simulink model "three_level_sv"  (R2025a)
settings: Solver=ode1be  StartTime=0.0  StopTime=simlength  FixedStep=ts_sim  MaxStep=ts_sim
undefined symbols (not defined in the file): number_of_cells, Q, q1Kalman, q2Kalman, q3Kalman, rKalman, tc, ts_afe, ts_zvs, tsample, Vbattery_nom
libraries: fl_lib x59, nesl_utility x30, ee_lib x1, lithium_ion_cell_lib x1, simulink x1
(part 2 of 2)

== system three_level_sv/theee-level-inverter/three-level-inverter/stage-1/three-level-inverter/switch_3 ==
  Diode : fl_lib/Electrical/Electrical Elements/Diode  Vf=Vdon_diode V  Ron=Rdon_diode Ohm  Goff=1e-8 1/Ohm  i_specify=off  i_priority=None  i=0 A  i_nominal_specify=off  i_nominal_value=1  i_nominal_unit=A  v_specify=off  v_priority=None  v=0 V  v_nominal_specify=off  v_nominal_value=1  v_nominal_unit=V
  Switch : fl_lib/Electrical/Electrical Elements/Switch  R_closed=Ron Ohm  G_open=1e-8 1/Ohm  Threshold=7.5  i_specify=off  i_priority=None  i=0 A  i_nominal_specify=off  i_nominal_value=1  i_nominal_unit=A  v_specify=off  v_priority=None  v=0 V  v_nominal_specify=off  v_nominal_value=1  v_nominal_unit=V
  G : PMIOPort  Side=Left
  C : PMIOPort  Port=2  Side=Left
  E : PMIOPort  Port=3  Side=Right
  connections:
  Diode/LConn1 -- E/RConn1 -- Switch/LConn1
  Switch/RConn1 -- G/RConn1
  Switch/RConn2 -- Diode/RConn1 -- C/RConn1

== system three_level_sv/theee-level-inverter/three-level-inverter/stage-1/three-level-inverter/switch_4 ==
  Diode : fl_lib/Electrical/Electrical Elements/Diode  Vf=Vdon_diode V  Ron=Rdon_diode Ohm  Goff=1e-8 1/Ohm  i_specify=off  i_priority=None  i=0 A  i_nominal_specify=off  i_nominal_value=1  i_nominal_unit=A  v_specify=off  v_priority=None  v=0 V  v_nominal_specify=off  v_nominal_value=1  v_nominal_unit=V
  Switch : fl_lib/Electrical/Electrical Elements/Switch  R_closed=Ron Ohm  G_open=1e-8 1/Ohm  Threshold=7.5  i_specify=off  i_priority=None  i=0 A  i_nominal_specify=off  i_nominal_value=1  i_nominal_unit=A  v_specify=off  v_priority=None  v=0 V  v_nominal_specify=off  v_nominal_value=1  v_nominal_unit=V
  G : PMIOPort  Side=Left
  C : PMIOPort  Port=2  Side=Left
  E : PMIOPort  Port=3  Side=Right
  connections:
  C/RConn1 -- Diode/RConn1 -- Switch/RConn2
  Switch/RConn1 -- G/RConn1
  Switch/LConn1 -- E/RConn1 -- Diode/LConn1

== system three_level_sv/theee-level-inverter/three-level-inverter/stage-1/three-level-inverter/switch_5 ==
  Diode : fl_lib/Electrical/Electrical Elements/Diode  Vf=Vdon_diode V  Ron=Rdon_diode Ohm  Goff=1e-8 1/Ohm  i_specify=off  i_priority=None  i=0 A  i_nominal_specify=off  i_nominal_value=1  i_nominal_unit=A  v_specify=off  v_priority=None  v=0 V  v_nominal_specify=off  v_nominal_value=1  v_nominal_unit=V
  Switch : fl_lib/Electrical/Electrical Elements/Switch  R_closed=Ron Ohm  G_open=1e-8 1/Ohm  Threshold=7.5  i_specify=off  i_priority=None  i=0 A  i_nominal_specify=off  i_nominal_value=1  i_nominal_unit=A  v_specify=off  v_priority=None  v=0 V  v_nominal_specify=off  v_nominal_value=1  v_nominal_unit=V
  G : PMIOPort  Side=Left
  C : PMIOPort  Port=2  Side=Left
  E : PMIOPort  Port=3  Side=Right
  connections:
  Diode/LConn1 -- E/RConn1 -- Switch/LConn1
  Switch/RConn1 -- G/RConn1
  Switch/RConn2 -- Diode/RConn1 -- C/RConn1

== system three_level_sv/theee-level-inverter/three-level-inverter/stage-1/three-level-inverter/switch_6 ==
  Diode : fl_lib/Electrical/Electrical Elements/Diode  Vf=Vdon_diode V  Ron=Rdon_diode Ohm  Goff=1e-8 1/Ohm  i_specify=off  i_priority=None  i=0 A  i_nominal_specify=off  i_nominal_value=1  i_nominal_unit=A  v_specify=off  v_priority=None  v=0 V  v_nominal_specify=off  v_nominal_value=1  v_nominal_unit=V
  Switch : fl_lib/Electrical/Electrical Elements/Switch  R_closed=Ron Ohm  G_open=1e-8 1/Ohm  Threshold=7.5  i_specify=off  i_priority=None  i=0 A  i_nominal_specify=off  i_nominal_value=1  i_nominal_unit=A  v_specify=off  v_priority=None  v=0 V  v_nominal_specify=off  v_nominal_value=1  v_nominal_unit=V
  G : PMIOPort  Side=Left
  C : PMIOPort  Port=2  Side=Left
  E : PMIOPort  Port=3  Side=Right
  connections:
  C/RConn1 -- Diode/RConn1 -- Switch/RConn2
  Switch/RConn1 -- G/RConn1
  Switch/LConn1 -- E/RConn1 -- Diode/LConn1

== system three_level_sv/theee-level-inverter/three-level-inverter/stage-1/three-level-inverter/switch_7 ==
  Diode : fl_lib/Electrical/Electrical Elements/Diode  Vf=Vdon_diode V  Ron=Rdon_diode Ohm  Goff=1e-8 1/Ohm  i_specify=off  i_priority=None  i=0 A  i_nominal_specify=off  i_nominal_value=1  i_nominal_unit=A  v_specify=off  v_priority=None  v=0 V  v_nominal_specify=off  v_nominal_value=1  v_nominal_unit=V
  Switch : fl_lib/Electrical/Electrical Elements/Switch  R_closed=Ron Ohm  G_open=1e-8 1/Ohm  Threshold=7.5  i_specify=off  i_priority=None  i=0 A  i_nominal_specify=off  i_nominal_value=1  i_nominal_unit=A  v_specify=off  v_priority=None  v=0 V  v_nominal_specify=off  v_nominal_value=1  v_nominal_unit=V
  G : PMIOPort  Side=Left
  C : PMIOPort  Port=2  Side=Left
  E : PMIOPort  Port=3  Side=Right
  connections:
  Diode/LConn1 -- E/RConn1 -- Switch/LConn1
  Switch/RConn1 -- G/RConn1
  Switch/RConn2 -- Diode/RConn1 -- C/RConn1

== system three_level_sv/theee-level-inverter/three-level-inverter/stage-1/three-level-inverter/switch_8 ==
  Diode : fl_lib/Electrical/Electrical Elements/Diode  Vf=Vdon_diode V  Ron=Rdon_diode Ohm  Goff=1e-8 1/Ohm  i_specify=off  i_priority=None  i=0 A  i_nominal_specify=off  i_nominal_value=1  i_nominal_unit=A  v_specify=off  v_priority=None  v=0 V  v_nominal_specify=off  v_nominal_value=1  v_nominal_unit=V
  Switch : fl_lib/Electrical/Electrical Elements/Switch  R_closed=Ron Ohm  G_open=1e-8 1/Ohm  Threshold=7.5  i_specify=off  i_priority=None  i=0 A  i_nominal_specify=off  i_nominal_value=1  i_nominal_unit=A  v_specify=off  v_priority=None  v=0 V  v_nominal_specify=off  v_nominal_value=1  v_nominal_unit=V
  G : PMIOPort  Side=Left
  C : PMIOPort  Port=2  Side=Left
  E : PMIOPort  Port=3  Side=Right
  connections:
  C/RConn1 -- Diode/RConn1 -- Switch/RConn2
  Switch/RConn1 -- G/RConn1
  Switch/LConn1 -- E/RConn1 -- Diode/LConn1

== system three_level_sv/theee-level-inverter/three-level-inverter/stage-1/three-level-inverter/switch_9 ==
  Diode : fl_lib/Electrical/Electrical Elements/Diode  Vf=Vdon_diode V  Ron=Rdon_diode Ohm  Goff=1e-8 1/Ohm  i_specify=off  i_priority=None  i=0 A  i_nominal_specify=off  i_nominal_value=1  i_nominal_unit=A  v_specify=off  v_priority=None  v=0 V  v_nominal_specify=off  v_nominal_value=1  v_nominal_unit=V
  Switch : fl_lib/Electrical/Electrical Elements/Switch  R_closed=Ron Ohm  G_open=1e-8 1/Ohm  Threshold=7.5  i_specify=off  i_priority=None  i=0 A  i_nominal_specify=off  i_nominal_value=1  i_nominal_unit=A  v_specify=off  v_priority=None  v=0 V  v_nominal_specify=off  v_nominal_value=1  v_nominal_unit=V
  G : PMIOPort  Side=Left
  C : PMIOPort  Port=2  Side=Left
  E : PMIOPort  Port=3  Side=Right
  connections:
  Diode/LConn1 -- E/RConn1 -- Switch/LConn1
  Switch/RConn1 -- G/RConn1
  Switch/RConn2 -- Diode/RConn1 -- C/RConn1

== matlab function three_level_sv/theee-level-inverter/pwm_commands/abc2alphabeta ==
  data: u input; alpha output; v input; w input; beta output
function [alpha,beta] = abc2alphabeta(u, v, w)

    alpha = 2/3 * (u - 1/2 * v - 1/2 * w);
    beta = 2/3 * (sqrt(3)/2 * v - sqrt(3)/2 * w);

end

== matlab function three_level_sv/theee-level-inverter/pwm_commands/counter_6 ==
  data: y output; Nmax parameter
function y = count_index(Nmax)

coder.extrinsic('evalin'); 

persistent x
    if isempty(x)
        x = 1;
    end

    if (x >= Nmax)
        x = 1;
    else
        x = x + 1;
    end


    if (x >= Nmax)
        y = Nmax;
    elseif (x <= 1)
        y = 1;
    else
        y = x;
    end
end

== matlab function three_level_sv/theee-level-inverter/pwm_commands/index2sv_6 ==
  data: i input; y output
function y = inner_sv_index(i)

    if (i == 1)
        y = [1 0 0]; 
    elseif (i == 2)
        y = [1 1 0]; 
    elseif (i == 3)
        y = [0 1 0]; 
    elseif (i == 4)
        y = [0 1 1]; 
    elseif (i == 5)
        y = [0 0 1];     
    elseif (i == 6)
        y = [1 0 1]; 
    else
        y = [0 0 0];
    end
end

== matlab function three_level_sv/theee-level-inverter/pwm_commands/index2sv_12 ==
  data: i input; y output
function y = outer_sv_index(i)

    if (i == 1)
        y = [1 -1 -1]; 
    elseif (i == 2)
        y = [1 0 -1]; 
    elseif (i == 3)
        y = [1 1 -1]; 
    elseif (i == 4)
        y = [0 1 -1]; 
    elseif (i == 5)
        y = [-1 1 -1];     
    elseif (i == 6)
        y = [-1 1 0]; 
    elseif (i == 7)
        y = [-1 1 1]; 
    elseif (i == 8)
        y = [-1 0 1]; 
    elseif (i == 9)
        y = [-1 -1 1]; 
    elseif (i == 10)
        y = [0 -1 1];
    elseif (i == 11)
        y = [1 -1 1]; 
    elseif (i == 12)
        y = [1 -1 0]; 
    else
        y = [0 0 0];
    end
end

== matlab function three_level_sv/theee-level-inverter/pwm_commands/sv2gata_cmds ==
  data: u input; y output
function y = three_level_sv(u)

u_nnn = [-1 -1 -1];
u_nno = [-1 -1 0];
u_nnp = [-1 -1 1];

u_non = [-1 0 -1];
u_noo = [-1 0 0];
u_nop = [-1 0 1];

u_npn = [-1 1 -1];
u_npo = [-1 1 0];
u_npp = [-1 1 1];

u_onn = [0 -1 -1];
u_ono = [0 -1 0];
u_onp = [0 -1 1];

u_oon = [0 0 -1];
u_ooo = [0 0 0];
u_oop = [0 0 1];

u_opn = [0 1 -1];
u_opo = [0 1 0];
u_opp = [0 1 1];

u_pnn = [1 -1 -1];
u_pno = [1 -1 0];
u_pnp = [1 -1 1];

u_pon = [1 0 -1];
u_poo = [1 0 0];
u_pop = [1 0 1];

u_ppn = [1 1 -1];
u_ppo = [1 1 0];
u_ppp = [1 1 1];

u_nnn_g = [0 0 1 1 0 0 1 1 0 0 1 1];
u_nno_g = [0 0 1 1 0 0 1 1 0 1 1 0];
u_nnp_g = [0 0 1 1 0 0 1 1 1 1 0 0];

u_non_g = [0 0 1 1 0 1 1 0 0 0 1 1];
u_noo_g = [0 0 1 1 0 1 1 0 0 1 1 0];
u_nop_g = [0 0 1 1 0 1 1 0 1 1 0 0];

u_npn_g = [0 0 1 1 1 1 0 0 0 0 1 1];
u_npo_g = [0 0 1 1 1 1 0 0 0 1 1 0];
u_npp_g = [0 0 1 1 1 1 0 0 1 1 0 0];

u_onn_g = [0 1 1 0 0 0 1 1 0 0 1 1];
u_ono_g = [0 1 1 0 0 0 1 1 0 1 1 0];
u_onp_g = [0 1 1 0 0 0 1 1 1 1 0 0];

u_oon_g = [0 1 1 0 0 1 1 0 0 0 1 1];
u_ooo_g = [0 1 1 0 0 1 1 0 0 1 1 0];
u_oop_g = [0 1 1 0 0 1 1 0 1 1 0 0];

u_opn_g = [0 1 1 0 1 1 0 0 0 0 1 1];
u_opo_g = [0 1 1 0 1 1 0 0 0 1 1 0];
u_opp_g = [0 1 1 0 1 1 0 0 1 1 0 0];

u_pnn_g = [1 1 0 0 0 0 1 1 0 0 1 1];
u_pno_g = [1 1 0 0 0 0 1 1 0 1 1 0];
u_pnp_g = [1 1 0 0 0 0 1 1 1 1 0 0];

u_pon_g = [1 1 0 0 0 1 1 0 0 0 1 1];
u_poo_g = [1 1 0 0 0 1 1 0 0 1 1 0];
u_pop_g = [1 1 0 0 0 1 1 0 1 1 0 0];

u_ppn_g = [1 1 0 0 1 1 0 0 0 0 1 1];
u_ppo_g = [1 1 0 0 1 1 0 0 0 1 1 0];
u_ppp_g = [1 1 0 0 1 1 0 0 1 1 0 0];

if (u == u_nnn)
y = u_nnn_g;
elseif (u == u_nno)
y = u_nno_g;
elseif (u == u_nnp)
y = u_nnp_g;
elseif (u == u_non)
y = u_non_g;
elseif (u == u_noo)
y = u_noo_g;
elseif (u == u_nop)
y = u_nop_g;
elseif (u == u_npn)
y = u_npn_g;
elseif (u == u_npo)
y = u_npo_g;
elseif (u == u_npp)
y = u_npp_g;
elseif (u == u_onn)
y = u_onn_g;
elseif (u == u_ono)
y = u_ono_g;
elseif (u == u_onp)
y = u_onp_g;
elseif (u == u_oon)
y = u_oon_g;
elseif (u == u_ooo)
y = u_ooo_g;
elseif (u == u_oop)
y = u_oop_g;
elseif (u == u_opn)
y = u_opn_g;
elseif (u == u_opo)
y = u_opo_g;
elseif (u == u_opp)
y = u_opp_g;
elseif (u == u_pnn)
y = u_pnn_g;
elseif (u == u_pno)
y = u_pno_g;
elseif (u == u_pnp)
y = u_pnp_g;
elseif (u == u_pon)
y = u_pon_g;
elseif (u == u_poo)
y = u_poo_g;
elseif (u == u_pop)
y = u_pop_g;
elseif (u == u_ppn)
y = u_ppn_g;
elseif (u == u_ppo)
y = u_ppo_g;
elseif (u == u_ppp)
y = u_ppp_g;
else
   y = u_ooo_g; 
end

== matlab function three_level_sv/theee-level-inverter/battery_system/LithiumIonBattery/SOC_estimator/Kalman_observer/kalman_observer_gains ==
  data: i input; ts input; l1 output; z input; q1 input; q2 input; q3 input; r input; Q input; l2 output; l3 output
function [l1,l2,l3] = EKF(i,ts,z,q1,q2,q3,r,Q)

    persistent  p11 p12 p13 p21 p22 p23 p31 p32 p33

    if isempty(p11)
        p11 = q1;
        p12 = 0;
        p13 = 0;
        p21 = 0;
        p22 = q2;
        p23 = 0;
        p31 = 0;
        p32 = 0;
        p33 = q3;
    end
    R = 0.15;
    C = 10;
    M = 125;
    E_1 = -1.031;
    E1 = 0.2156;
    E2 = 0;
    E3 = 0;
    Elog = -0.05;
    alpha = 35;

    a11 = 1;
    a12 = 0;
    a13 = 0;
    a21 = 0;
    a22 = exp(-ts/(R*C));
    a23 = 0;
    a31 = 0;
    a32 = 0;
    a33 = abs(exp(-i*ts/Q));

    c1 = -alpha*E_1*abs(exp(-alpha*z)) + E1 + 2*E2*z + 3*E3*z^2 - Elog/(1-z+ts);
    c2 = -R;
    c3 = M;
    
    p11_pr = a11*(a11*p11 + a12*p21 + a13*p31) + a12*(a11*p12 + a12*p22 + a13*p32) + a13*(a11*p13 + a12*p23 + a13*p33) + q1;

    p12_pr = a21*(a11*p11 + a12*p21 + a13*p31) + a22*(a11*p12 + a12*p22 + a13*p32) + a23*(a11*p13 + a12*p23 + a13*p33);

    p13_pr = a31*(a11*p11 + a12*p21 + a13*p31) + a32*(a11*p12 + a12*p22 + a13*p32) + a33*(a11*p13 + a12*p23 + a13*p33);

    p21_pr = a11*(a21*p11 + a22*p21 + a23*p31) + a12*(a21*p12 + a22*p22 + a23*p32) + a13*(a21*p13 + a22*p23 + a23*p33);

    p22_pr = a21*(a21*p11 + a22*p21 + a23*p31) + a22*(a21*p12 + a22*p22 + a23*p32) + a23*(a21*p13 + a22*p23 + a23*p33) + q2;

    p23_pr = a31*(a21*p11 + a22*p21 + a23*p31) + a32*(a21*p12 + a22*p22 + a23*p32) + a33*(a21*p13 + a22*p23 + a23*p33);

    p31_pr = a11*(a31*p11 + a32*p21 + a33*p31) + a12*(a31*p12 + a32*p22 + a33*p32) + a13*(a31*p13 + a32*p23 + a33*p33);

    p32_pr = a21*(a31*p11 + a32*p21 + a33*p31) + a22*(a31*p12 + a32*p22 + a33*p32) + a23*(a31*p13 + a32*p23 + a33*p33);

    p33_pr = a31*(a31*p11 + a32*p21 + a33*p31) + a32*(a31*p12 + a32*p22 + a33*p32) + a33*(a31*p13 + a32*p23 + a33*p33) + q3;

    den = c1*(c1*p11 + c2*p21 + c3*p31) + c2*(c1*p12 + c2*p22 + c3*p32) + c3*(c1*p13 + c2*p23 + c3*p33) + r;
 
    l1 = (c1*p11 + c2*p12 + c3*p13)/den;
    l2 = (c1*p21 + c2*p22 + c3*p23)/den;
    l3 = (c1*p31 + c2*p32 + c3*p33)/den;
    
    p11 = (1 - c1*l1)*p11_pr - c2*l1*p21_pr - c3*l1*p31_pr;
    
    p12 = (1 - c1*l1)*p12_pr - c2*l1*p22_pr - c3*l1*p32_pr;
    
    p13 = (1 - c1*l1)*p13_pr - c2*l1*p23_pr - c3*l1*p33_pr;
    
    p21 = -c1*l2*p11_pr + (1 - c2*l2)*p21_pr - c3*l2*p31_pr;
    
    p22 = -c1*l2*p12_pr + (1 - c2*l2)*p22_pr - c3*l2*p32_pr;
    
    p23 = -c1*l2*p13_pr + (1 - c2*l2)*p23_pr - c3*l2*p33_pr;
    
    p31 = -c1*l3*p11_pr - c2*l3*p21_pr + (1 - c3*l3)*p31_pr;
    
    p32 = -c1*l3*p12_pr - c2*l3*p22_pr + (1 - c3*l3)*p32_pr;
    
    p33 = -c1*l3*p13_pr - c2*l3*p23_pr + (1 - c3*l3)*p33_pr;
end

== matlab function three_level_sv/theee-level-inverter/pwm_commands/counter_12 ==
  data: y output; Nmax parameter
function y = count_index(Nmax)

coder.extrinsic('evalin'); 

persistent x
    if isempty(x)
        x = 1;
    end

    if (x >= Nmax)
        x = 1;
    else
        x = x + 1;
    end


    if (x >= Nmax)
        y = Nmax;
    elseif (x <= 1)
        y = 1;
    else
        y = x;
    end
end

== matlab function three_level_sv/theee-level-inverter/battery_system/LithiumIonBattery/SOC_estimator/Kalman_observer/lithium-ion battery model ==
  data: i input; SOC output; u output; ts input; Q input; l1 input; l2 input; l3 input; vout input; x output
function [SOC, u, x] = lithium_ion_battery(i,ts,Q,l1,l2,l3,vout)

    persistent z_po ir_po h_po vout_hat

    if isempty(z_po)
        ir_po = 0;
        h_po = 0;
        z_po = 0.35;        
    end
    
        R0 = 0.15;
        R = 0.15;
        C = 0.1;
        M = 125;
        E_1 = -1.031;
        E0 = 3.685;
        E1 = 0.2156;
        E2 = 0;
        E3 = 0;
        Elog = -0.05;
        alpha = 35;
        N = 100;
        
        z_pr = z_po - ts/Q*i ;
    
        ir_pr = exp(-ts/(R*C))*ir_po + (1-exp(-ts/(R*C)))*i;

        h_pr = exp(-abs(i)*ts/Q)*h_po - (1-exp(-abs(i)*ts/Q))*sign(i);
        
        OCV = E_1*exp(-z_pr*alpha) + E0 + E1*z_pr + E2*z_pr^2 + E3*z_pr^3 + Elog*log(1-z_pr+ts);
        
        vout_hat = OCV*N + M*h_pr - R*ir_pr - R0*i;
        
        z_po = z_pr + l1*(vout - vout_hat);
        ir_po = ir_pr + l2*(vout - vout_hat);
        h_po = h_pr + l3*(vout - vout_hat);
        u = vout_hat;
        
        x = [z_po; ir_po; h_po];

    SOC = z_po;
end
